simulink model "actuator_control"  (R2016b)
settings: configuration reference "Configuration4khz" (kept outside this file)
values from neighbouring files (symbols this model uses):
  sample_time = 0.0005    [ElmoIncremental.m]
undefined symbols (not defined in the file or in its folder): A_kalman_sea_swing_back, A_kalman_sea_swing_front, A_kalman_swing_load, A_lpf_1to4, A_lpf_dtau, A_lpf_sea_kalman_velocities, B1_lpf_1to4, B1_lpf_dtau, B1_lpf_sea_kalman_velocities, B2_lpf_1to4, B2_lpf_dtau, B2_lpf_sea_kalman_velocities, B_kalman_sea_swing_back, B_kalman_sea_swing_front, B_kalman_swing_load, C_kalman_sea_swing, C_kalman_swing_load, DiscIntNeverNeededParam, Discrete, elmo_sample_time, fdesignblkfcn, gcbh, initial_dx_estimate, j_segments, k_sea_low, kalman_load_to_deflect_transmission, lateral_motor_efficiency, LEG_MTR_GEAR_RATIO, P0_kalman_sea_swing, P0_kalman_swing_load, Q_kalman_load_torque, Q_kalman_rotor_torque, Q_kalman_trunk_torque, R_kalman_absolute_fail, R_kalman_absolute_normal, R_kalman_incremental_loaded, R_kalman_incremental_unloaded, sea_kalman_sample_time, swing_collision_damping_rate, Time
libraries: simulink x17, ctrlSharedLib x8, dsparch4 x5, dspfdesign x1
(part 2 of 3)

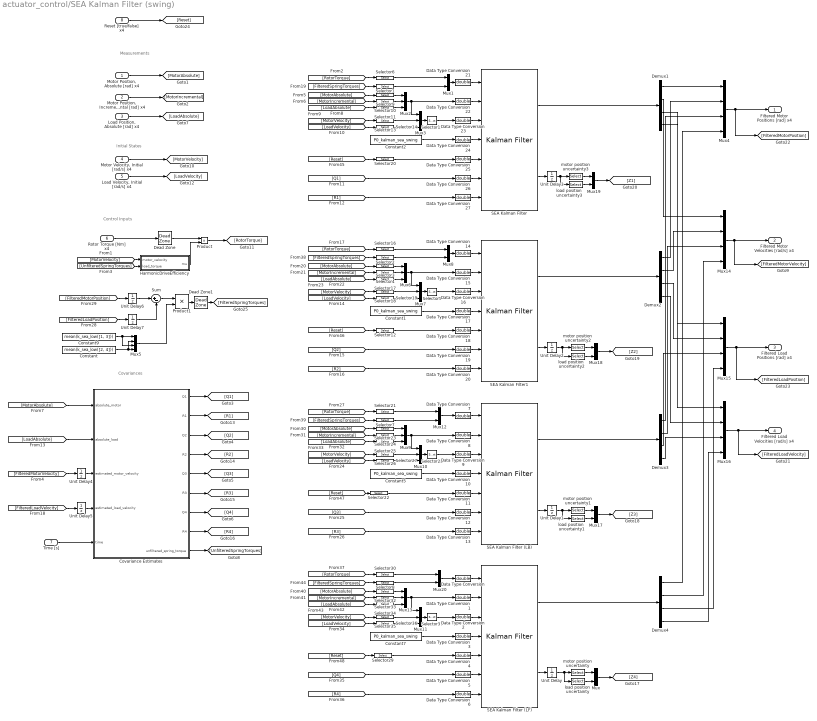
== system actuator_control/SEA Kalman Filter (swing) ==
  note: Measurements
  note: Control Inputs
  note: Initial States
  note: Covariances
  "Motor Position, Absolute [rad] x4" : Inport
  "Motor Position, Incremental [rad] x4" : Inport  Port=2
  "Load Position, Absolute [rad] x4" : Inport  Port=3
  "Motor Velocity, Initial [rad/s] x4" : Inport  Port=4
  "Load Velocity, Initial [rad/s] x4" : Inport  Port=5
  Rotor Torque [Nm] x4 : Inport  Port=6
  Time [s] : Inport  Port=7
  Reset [true/false] x4 : Inport  Port=8
  Constant : Constant  Value=mean(k_sea_low([2, 4]))
  Constant{1..2,5,7} (4 alike) : Constant  Value=P0_kalman_sea_swing
  Constant9 : Constant  Value=mean(k_sea_low([1, 3]))
  Covariance Estimates : MATLAB Function  TreatAsAtomicUnit=on
  Data Type Conversion{,1..27} (28 alike) : DataTypeConversion  OutDataTypeStr=double
  Dead Zone : DeadZone  LowerValue=-30/50  UpperValue=30/50  SaturateOnIntegerOverflow=on
  Dead Zone1 : DeadZone  LowerValue=-2.5  UpperValue=2.5  SaturateOnIntegerOverflow=on
  Demux{1..4} (4 alike) : Demux
  HarmonicDriveEfficiency : MATLAB Function  TreatAsAtomicUnit=on
  Mux{,1,8,12,17..20} (8 alike) : Mux  Inputs=2
  Mux{2..3,6..7,9..11,13} (8 alike) : Mux  Inputs=3
  Mux{4..5,14..16} (5 alike) : Mux
  Product : Product
  Product1 : Product
  SEA Kalman Filter : ctrlSharedLib/Kalman Filter  TimeDomain=Discrete-Time  UseCurrentEstimator=on  ModelSource=Individual A, B, C, D matrices  ModelSourceVariable=A_kf  A=A_kalman_sea_swing_back  B=B_kalman_sea_swing_back  C=C_kalman_sea_swing  D=0  NumberOfStates=2  NumberOfInputs=1  NumberOfOutputs=2  InitialEstimateSource=Input port  X0=initial_dx_estimate  P0=P0_kalman_transverse  UseK=off  UseGH=on  NumberOfProcessNoiseInputs=1  G=G_kalman_sea_swing_back  TimeInvariantG=on  H=0  TimeInvariantH=on  Q=1  TimeInvariantQ=off  R=1  TimeInvariantR=off  N=0  TimeInvariantN=on  AddInputPort=on  AddEnablePort=off  ExternalReset=Rising  OutputEstimatedY=off  OutputP=on  Ts=sea_kalman_sample_time
  SEA Kalman Filter (LB) : ctrlSharedLib/Kalman Filter  TimeDomain=Discrete-Time  UseCurrentEstimator=on  ModelSource=Individual A, B, C, D matrices  ModelSourceVariable=A_kf  A=A_kalman_sea_swing_back  B=B_kalman_sea_swing_back  C=C_kalman_sea_swing  D=0  NumberOfStates=2  NumberOfInputs=1  NumberOfOutputs=2  InitialEstimateSource=Input port  X0=initial_dx_estimate  P0=P0_kalman_transverse  UseK=off  UseGH=on  NumberOfProcessNoiseInputs=1  G=G_kalman_sea_swing_back  TimeInvariantG=on  H=0  TimeInvariantH=on  Q=1  TimeInvariantQ=off  R=1  TimeInvariantR=off  N=0  TimeInvariantN=on  AddInputPort=on  AddEnablePort=off  ExternalReset=Rising  OutputEstimatedY=off  OutputP=on  Ts=sea_kalman_sample_time
  SEA Kalman Filter (LF) : ctrlSharedLib/Kalman Filter  TimeDomain=Discrete-Time  UseCurrentEstimator=on  ModelSource=Individual A, B, C, D matrices  ModelSourceVariable=A_kf  A=A_kalman_sea_swing_front  B=B_kalman_sea_swing_front  C=C_kalman_sea_swing  D=0  NumberOfStates=2  NumberOfInputs=1  NumberOfOutputs=2  InitialEstimateSource=Input port  X0=initial_dx_estimate  P0=P0_kalman_transverse  UseK=off  UseGH=on  NumberOfProcessNoiseInputs=1  G=G_kalman_sea_swing_front  TimeInvariantG=on  H=0  TimeInvariantH=on  Q=1  TimeInvariantQ=off  R=1  TimeInvariantR=off  N=0  TimeInvariantN=on  AddInputPort=on  AddEnablePort=off  ExternalReset=Rising  OutputEstimatedY=off  OutputP=on  Ts=sea_kalman_sample_time
  SEA Kalman Filter1 : ctrlSharedLib/Kalman Filter  TimeDomain=Discrete-Time  UseCurrentEstimator=on  ModelSource=Individual A, B, C, D matrices  ModelSourceVariable=A_kf  A=A_kalman_sea_swing_front  B=B_kalman_sea_swing_front  C=C_kalman_sea_swing  D=0  NumberOfStates=2  NumberOfInputs=1  NumberOfOutputs=2  InitialEstimateSource=Input port  X0=initial_dx_estimate  P0=P0_kalman_transverse  UseK=off  UseGH=on  NumberOfProcessNoiseInputs=1  G=G_kalman_sea_swing_front  TimeInvariantG=on  H=0  TimeInvariantH=on  Q=1  TimeInvariantQ=off  R=1  TimeInvariantR=off  N=0  TimeInvariantN=on  AddInputPort=on  AddEnablePort=off  ExternalReset=Rising  OutputEstimatedY=off  OutputP=on  Ts=sea_kalman_sample_time
  Selector{1,6,9..11,13..14,20} (8 alike) : Selector  InputPortWidth=4  IndexOptions=Index vector (dialog)  Indices=[1]  OutputSizes=1
  Selector{2..4,12,16..19} (8 alike) : Selector  InputPortWidth=4  IndexOptions=Index vector (dialog)  Indices=[2]  OutputSizes=1
  Selector{5,15,28,37} (4 alike) : Selector  InputPortWidth=5  IndexOptions=Index vector (dialog)  Indices=[1 4 3 5]  OutputSizes=1
  Selector{7,21..27} (8 alike) : Selector  InputPortWidth=4  IndexOptions=Index vector (dialog)  Indices=[3]  OutputSizes=1
  Selector{8,29..30,32..36} (8 alike) : Selector  InputPortWidth=4  IndexOptions=Index vector (dialog)  Indices=[4]  OutputSizes=1
  Sum : Sum  Inputs=|+-
  Unit Delay{,1..7} (8 alike) : UnitDelay  SampleTime=-1
  load position uncertainty{,1..3} (4 alike) : Selector  NumberOfDimensions=2  InputPortWidth=2  IndexOptions=Index vector (dialog),Index vector (dialog)  Indices=[3],[3]  OutputSizes=1,1
  motor position uncertainty{,1..3} (4 alike) : Selector  NumberOfDimensions=2  InputPortWidth=2  IndexOptions=Index vector (dialog),Index vector (dialog)  Indices=[1],[1]  OutputSizes=1,1
  Filtered Motor Positions [rad] x4 : Outport
  Filtered Motor Velocities [rad/s] x4 : Outport  Port=2
  Filtered Load Positions [rad] x4 : Outport  Port=3
  Filtered Load Velocities [rad/s] x4 : Outport  Port=4
  wires:
  "Motor Position, Incremental [rad] x4"/1 -> [MotorIncremental]
  "Motor Position, Absolute [rad] x4"/1 -> [MotorAbsolute]
  "Load Position, Absolute [rad] x4"/1 -> [LoadAbsolute]
  Mux2/1 -> Mux3/1, Data Type Conversion22/1
  Selector6/1 -> Mux1/1
  [RotorTorque] -> Selector6/1
  Selector11/1 -> Mux2/3
  Selector10/1 -> Mux2/2
  Selector9/1 -> Mux2/1
  [MotorAbsolute] -> Selector9/1
  [MotorIncremental] -> Selector10/1
  [LoadAbsolute] -> Selector11/1
  "Motor Velocity, Initial [rad/s] x4"/1 -> [MotorVelocity]
  "Load Velocity, Initial [rad/s] x4"/1 -> [LoadVelocity]
  Mux3/1 -> Selector15/1
  [MotorVelocity] -> Selector13/1
  [LoadVelocity] -> Selector14/1
  Selector14/1 -> Mux3/3
  Selector13/1 -> Mux3/2
  Selector15/1 -> Data Type Conversion23/1
  Constant2/1 -> Data Type Conversion24/1
  [Reset] -> Selector20/1
  [R1] -> Data Type Conversion27/1
  [Q1] -> Data Type Conversion26/1
  SEA Kalman Filter/1 -> Demux1/1
  Covariance Estimates/1(Q1) -> [Q1]
  Covariance Estimates/3(Q2) -> [Q2]
  Covariance Estimates/5(Q3) -> [Q3]
  Covariance Estimates/7(Q4) -> [Q4]
  Covariance Estimates/2(R1) -> [R1]
  Covariance Estimates/4(R2) -> [R2]
  Covariance Estimates/6(R3) -> [R3]
  Covariance Estimates/8(R4) -> [R4]
  Mux6/1 -> Data Type Conversion15/1, Mux7/1
  [RotorTorque] -> Selector16/1
  Selector17/1 -> Mux6/3
  Selector4/1 -> Mux6/2
  Selector3/1 -> Mux6/1
  [MotorAbsolute] -> Selector3/1
  [MotorIncremental] -> Selector4/1
  [LoadAbsolute] -> Selector17/1
  Mux7/1 -> Selector5/1
  [MotorVelocity] -> Selector18/1
  [LoadVelocity] -> Selector19/1
  Selector19/1 -> Mux7/3
  Selector18/1 -> Mux7/2
  Selector5/1 -> Data Type Conversion16/1
  Constant1/1 -> Data Type Conversion17/1
  [Reset] -> Selector12/1
  [R2] -> Data Type Conversion20/1
  [Q2] -> Data Type Conversion19/1
  SEA Kalman Filter1/1 -> Demux2/1
  Mux9/1 -> Mux10/1, Data Type Conversion8/1
  [RotorTorque] -> Selector21/1
  Selector25/1 -> Mux9/3
  Selector24/1 -> Mux9/2
  Selector23/1 -> Mux9/1
  [MotorAbsolute] -> Selector23/1
  [MotorIncremental] -> Selector24/1
  [LoadAbsolute] -> Selector25/1
  Mux10/1 -> Selector28/1
  [MotorVelocity] -> Selector26/1
  [LoadVelocity] -> Selector27/1
  Selector27/1 -> Mux10/3
  Selector26/1 -> Mux10/2
  Selector28/1 -> Data Type Conversion9/1
  Constant5/1 -> Data Type Conversion10/1
  [Reset] -> Selector22/1
  [R3] -> Data Type Conversion13/1
  [Q3] -> Data Type Conversion12/1
  SEA Kalman Filter (LB)/1 -> Demux3/1
  Mux13/1 -> Data Type Conversion1/1, Mux11/1
  [RotorTorque] -> Selector30/1
  Selector34/1 -> Mux13/3
  Selector33/1 -> Mux13/2
  Selector32/1 -> Mux13/1
  [MotorAbsolute] -> Selector32/1
  [MotorIncremental] -> Selector33/1
  [LoadAbsolute] -> Selector34/1
  Mux11/1 -> Selector37/1
  [MotorVelocity] -> Selector35/1
  [LoadVelocity] -> Selector36/1
  Selector36/1 -> Mux11/3
  Selector35/1 -> Mux11/2
  Selector37/1 -> Data Type Conversion2/1
  Constant7/1 -> Data Type Conversion3/1
  [Reset] -> Selector29/1
  [R4] -> Data Type Conversion6/1
  [Q4] -> Data Type Conversion5/1
  SEA Kalman Filter (LF)/1 -> Demux4/1
  Demux1/1 -> Mux4/1
  Demux2/1 -> Mux4/2
  Demux3/1 -> Mux4/3
  Demux4/1 -> Mux4/4
  Demux1/2 -> Mux14/1
  Demux2/2 -> Mux14/2
  Demux3/2 -> Mux14/3
  Demux4/2 -> Mux14/4
  Demux1/3 -> Mux15/1
  Demux2/3 -> Mux15/2
  Demux3/3 -> Mux15/3
  Demux4/3 -> Mux15/4
  Demux1/4 -> Mux16/1
  Demux2/4 -> Mux16/2
  Demux3/4 -> Mux16/3
  Demux4/4 -> Mux16/4
  [LoadAbsolute] -> Covariance Estimates/2(absolute_load)
  [MotorAbsolute] -> Covariance Estimates/1(absolute_motor)
  SEA Kalman Filter (LF)/2 -> Unit Delay/1
  motor position uncertainty/1 -> Mux/1
  load position uncertainty/1 -> Mux/2
  Mux/1 -> [Z4]
  SEA Kalman Filter (LB)/2 -> Unit Delay1/1
  motor position uncertainty1/1 -> Mux17/1
  load position uncertainty1/1 -> Mux17/2
  Mux17/1 -> [Z3]
  SEA Kalman Filter1/2 -> Unit Delay2/1
  motor position uncertainty2/1 -> Mux18/1
  load position uncertainty2/1 -> Mux18/2
  Mux18/1 -> [Z2]
  SEA Kalman Filter/2 -> Unit Delay3/1
  motor position uncertainty3/1 -> Mux19/1
  load position uncertainty3/1 -> Mux19/2
  Mux19/1 -> [Z1]
  Unit Delay/1 -> load position uncertainty/1, motor position uncertainty/1
  Unit Delay1/1 -> load position uncertainty1/1, motor position uncertainty1/1
  Unit Delay2/1 -> motor position uncertainty2/1, load position uncertainty2/1
  Unit Delay3/1 -> load position uncertainty3/1, motor position uncertainty3/1
  Data Type Conversion/1 -> SEA Kalman Filter (LF)/1
  Data Type Conversion1/1 -> SEA Kalman Filter (LF)/2
  Data Type Conversion2/1 -> SEA Kalman Filter (LF)/3
  Data Type Conversion3/1 -> SEA Kalman Filter (LF)/4
  Data Type Conversion4/1 -> SEA Kalman Filter (LF)/5
  Data Type Conversion5/1 -> SEA Kalman Filter (LF)/6
  Data Type Conversion6/1 -> SEA Kalman Filter (LF)/7
  Data Type Conversion7/1 -> SEA Kalman Filter (LB)/1
  Data Type Conversion9/1 -> SEA Kalman Filter (LB)/3
  Data Type Conversion8/1 -> SEA Kalman Filter (LB)/2
  Data Type Conversion10/1 -> SEA Kalman Filter (LB)/4
  Data Type Conversion11/1 -> SEA Kalman Filter (LB)/5
  Data Type Conversion13/1 -> SEA Kalman Filter (LB)/7
  Data Type Conversion12/1 -> SEA Kalman Filter (LB)/6
  Data Type Conversion14/1 -> SEA Kalman Filter1/1
  Data Type Conversion15/1 -> SEA Kalman Filter1/2
  Data Type Conversion18/1 -> SEA Kalman Filter1/5
  Data Type Conversion19/1 -> SEA Kalman Filter1/6
  Data Type Conversion16/1 -> SEA Kalman Filter1/3
  Data Type Conversion17/1 -> SEA Kalman Filter1/4
  Data Type Conversion20/1 -> SEA Kalman Filter1/7
  Data Type Conversion21/1 -> SEA Kalman Filter/1
  Data Type Conversion25/1 -> SEA Kalman Filter/5
  Data Type Conversion24/1 -> SEA Kalman Filter/4
  Data Type Conversion23/1 -> SEA Kalman Filter/3
  Data Type Conversion26/1 -> SEA Kalman Filter/6
  Data Type Conversion22/1 -> SEA Kalman Filter/2
  Data Type Conversion27/1 -> SEA Kalman Filter/7
  Mux4/1 -> [FilteredMotorPosition], Filtered Motor Positions [rad] x4/1
  Mux15/1 -> [FilteredLoadPosition], Filtered Load Positions [rad] x4/1
  Mux14/1 -> [FilteredMotorVelocity], Filtered Motor Velocities [rad/s] x4/1
  Mux16/1 -> [FilteredLoadVelocity], Filtered Load Velocities [rad/s] x4/1
  HarmonicDriveEfficiency/1(mu) -> Product/2
  [MotorVelocity] -> HarmonicDriveEfficiency/1(motor_velocity)
  [UnfilteredSpringTorques] -> HarmonicDriveEfficiency/2(load_torque)
  Covariance Estimates/9(unfiltered_spring_torque) -> [UnfilteredSpringTorques]
  Time [s]/1 -> Covariance Estimates/5(time)
  [FilteredMotorVelocity] -> Unit Delay4/1
  [FilteredLoadVelocity] -> Unit Delay5/1
  Unit Delay4/1 -> Covariance Estimates/3(estimated_motor_velocity)
  Unit Delay5/1 -> Covariance Estimates/4(estimated_load_velocity)
  Rotor Torque [Nm] x4/1 -> Dead Zone/1
  Dead Zone/1 -> Product/1
  Mux1/1 -> Data Type Conversion21/1
  [FilteredSpringTorques] -> Selector1/1
  Selector1/1 -> Mux1/2
  [FilteredMotorPosition] -> Unit Delay6/1
  [FilteredLoadPosition] -> Unit Delay7/1
  Constant9/1 -> Mux5/1, Mux5/3
  Constant/1 -> Mux5/2, Mux5/4
  Sum/1 -> Product1/1
  Mux5/1 -> Product1/2
  Product1/1 -> Dead Zone1/1
  [FilteredSpringTorques] -> Selector2/1
  Selector2/1 -> Mux8/2
  Mux8/1 -> Data Type Conversion14/1
  Selector16/1 -> Mux8/1
  [FilteredSpringTorques] -> Selector7/1
  Selector7/1 -> Mux12/2
  Mux12/1 -> Data Type Conversion7/1
  Selector21/1 -> Mux12/1
  [FilteredSpringTorques] -> Selector8/1
  Selector8/1 -> Mux20/2
  Mux20/1 -> Data Type Conversion/1
  Selector30/1 -> Mux20/1
  Unit Delay7/1 -> Sum/2
  Unit Delay6/1 -> Sum/1
  Dead Zone1/1 -> [FilteredSpringTorques]
  Product/1 -> [RotorTorque]
  Reset [true/false] x4/1 -> [Reset]
  Selector12/1 -> Data Type Conversion18/1
  Selector20/1 -> Data Type Conversion25/1
  Selector22/1 -> Data Type Conversion11/1
  Selector29/1 -> Data Type Conversion4/1

== system actuator_control/Select Signal ==
  True/False x4 : Inport
  Signal True x4 : Inport  Port=2
  Signal False x4 : Inport  Port=3
  Demux : Demux
  Demux1 : Demux
  Demux2 : Demux
  Mux : Mux
  Switch{,1..3} (4 alike) : Switch  Criteria=u2 ~= 0
  Selected x4 : Outport
  wires:
  Mux/1 -> Selected x4/1
  True/False x4/1 -> Demux1/1
  Signal True x4/1 -> Demux/1
  Signal False x4/1 -> Demux2/1
  Demux/1 -> Switch/1
  Demux/2 -> Switch1/1
  Demux/3 -> Switch2/1
  Demux/4 -> Switch3/1
  Demux2/1 -> Switch/3
  Demux2/2 -> Switch1/3
  Demux2/3 -> Switch2/3
  Demux2/4 -> Switch3/3
  Demux1/1 -> Switch/2
  Demux1/2 -> Switch1/2
  Demux1/3 -> Switch2/2
  Demux1/4 -> Switch3/2
  Switch/1 -> Mux/1
  Switch1/1 -> Mux/2
  Switch2/1 -> Mux/3
  Switch3/1 -> Mux/4

== system actuator_control/Select Signal1 ==
  True/False x4 : Inport
  Signal True x4 : Inport  Port=2
  Signal False x4 : Inport  Port=3
  Demux : Demux
  Demux1 : Demux
  Demux2 : Demux
  Mux : Mux
  Switch{,1..3} (4 alike) : Switch  Criteria=u2 ~= 0
  Selected x4 : Outport
  wires:
  Switch3/1 -> Mux/4
  Switch2/1 -> Mux/3
  Switch1/1 -> Mux/2
  Switch/1 -> Mux/1
  Demux1/4 -> Switch3/2
  Demux1/3 -> Switch2/2
  Demux1/2 -> Switch1/2
  Demux1/1 -> Switch/2
  Demux2/4 -> Switch3/3
  Demux2/3 -> Switch2/3
  Demux2/2 -> Switch1/3
  Demux2/1 -> Switch/3
  Demux/4 -> Switch3/1
  Demux/3 -> Switch2/1
  Demux/2 -> Switch1/1
  Demux/1 -> Switch/1
  Signal False x4/1 -> Demux2/1
  Signal True x4/1 -> Demux/1
  True/False x4/1 -> Demux1/1
  Mux/1 -> Selected x4/1

== system actuator_control/Select Signal2 ==
  True/False x4 : Inport
  Signal True x4 : Inport  Port=2
  Signal False x4 : Inport  Port=3
  Demux : Demux
  Demux1 : Demux
  Demux2 : Demux
  Mux : Mux
  Switch{,1..3} (4 alike) : Switch  Criteria=u2 ~= 0
  Selected x4 : Outport
  wires:
  Mux/1 -> Selected x4/1
  True/False x4/1 -> Demux1/1
  Signal True x4/1 -> Demux/1
  Signal False x4/1 -> Demux2/1
  Demux/1 -> Switch/1
  Demux/2 -> Switch1/1
  Demux/3 -> Switch2/1
  Demux/4 -> Switch3/1
  Demux2/1 -> Switch/3
  Demux2/2 -> Switch1/3
  Demux2/3 -> Switch2/3
  Demux2/4 -> Switch3/3
  Demux1/1 -> Switch/2
  Demux1/2 -> Switch1/2
  Demux1/3 -> Switch2/2
  Demux1/4 -> Switch3/2
  Switch/1 -> Mux/1
  Switch1/1 -> Mux/2
  Switch2/1 -> Mux/3
  Switch3/1 -> Mux/4

== system actuator_control/Stance or Swing1 ==
  True/False x4 : Inport
  Signal True x4 : Inport  Port=2
  Signal False x4 : Inport  Port=3
  Demux : Demux
  Demux1 : Demux
  Demux2 : Demux
  Mux : Mux
  Switch{,1..3} (4 alike) : Switch  Criteria=u2 ~= 0
  Selected x4 : Outport
  wires:
  Switch3/1 -> Mux/4
  Switch2/1 -> Mux/3
  Switch1/1 -> Mux/2
  Switch/1 -> Mux/1
  Demux1/4 -> Switch3/2
  Demux1/3 -> Switch2/2
  Demux1/2 -> Switch1/2
  Demux1/1 -> Switch/2
  Demux2/4 -> Switch3/3
  Demux2/3 -> Switch2/3
  Demux2/2 -> Switch1/3
  Demux2/1 -> Switch/3
  Demux/4 -> Switch3/1
  Demux/3 -> Switch2/1
  Demux/2 -> Switch1/1
  Demux/1 -> Switch/1
  Signal False x4/1 -> Demux2/1
  Signal True x4/1 -> Demux/1
  True/False x4/1 -> Demux1/1
  Mux/1 -> Selected x4/1

== system actuator_control/Misc/Compare SEA Signals1 ==
  Finite Difference : Inport
  Kalman : Inport  Port=2
  Demux : Demux
  Demux1 : Demux
  Mux{6..9} (4 alike) : Mux  Inputs=2
  RB : Outport
  RF : Outport  Port=2
  LB : Outport  Port=3
  LF : Outport  Port=4
  wires:
  Demux/3 -> Mux8/1
  Demux/2 -> Mux7/1
  Demux1/1 -> Mux6/2
  Demux/1 -> Mux6/1
  Demux/4 -> Mux9/1
  Demux1/4 -> Mux9/2
  Kalman/1 -> Demux1/1
  Demux1/2 -> Mux7/2
  Finite Difference/1 -> Demux/1
  Demux1/3 -> Mux8/2
  Mux6/1 -> RB/1
  Mux7/1 -> RF/1
  Mux9/1 -> LF/1
  Mux8/1 -> LB/1

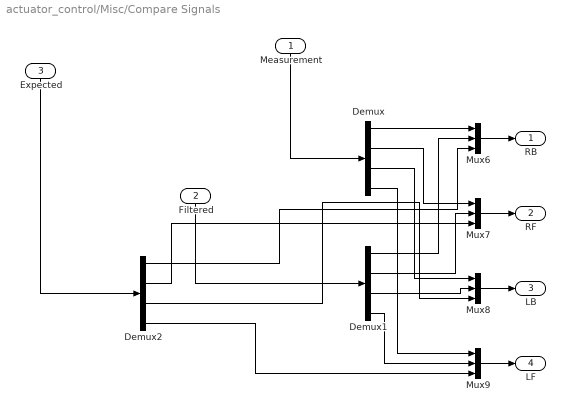
== system actuator_control/Misc/Compare Signals ==
  Measurement : Inport
  Filtered : Inport  Port=2
  Expected : Inport  Port=3
  Demux : Demux
  Demux1 : Demux
  Demux2 : Demux
  Mux{6..9} (4 alike) : Mux  Inputs=3
  RB : Outport
  RF : Outport  Port=2
  LB : Outport  Port=3
  LF : Outport  Port=4
  wires:
  Mux8/1 -> LB/1
  Mux9/1 -> LF/1
  Mux7/1 -> RF/1
  Mux6/1 -> RB/1
  Demux1/3 -> Mux8/2
  Measurement/1 -> Demux/1
  Demux1/2 -> Mux7/2
  Filtered/1 -> Demux1/1
  Demux1/4 -> Mux9/2
  Demux/4 -> Mux9/1
  Demux/1 -> Mux6/1
  Demux1/1 -> Mux6/2
  Demux/2 -> Mux7/1
  Demux/3 -> Mux8/1
  Expected/1 -> Demux2/1
  Demux2/1 -> Mux6/3
  Demux2/2 -> Mux7/3
  Demux2/3 -> Mux8/3
  Demux2/4 -> Mux9/3

== system actuator_control/Misc/Compare Torque Derivative Signals ==
  Measured : Inport
  Filtered : Inport  Port=2
  Expected : Inport  Port=3
  Demux : Demux
  Demux1 : Demux
  Demux2 : Demux
  Mux{6..9} (4 alike) : Mux  Inputs=3
  RB : Outport
  RF : Outport  Port=2
  LB : Outport  Port=3
  LF : Outport  Port=4
  wires:
  Demux2/4 -> Mux9/3
  Demux2/3 -> Mux8/3
  Demux2/2 -> Mux7/3
  Demux2/1 -> Mux6/3
  Expected/1 -> Demux2/1
  Demux/3 -> Mux8/1
  Demux/2 -> Mux7/1
  Demux1/1 -> Mux6/2
  Demux/1 -> Mux6/1
  Demux/4 -> Mux9/1
  Demux1/4 -> Mux9/2
  Filtered/1 -> Demux1/1
  Demux1/2 -> Mux7/2
  Measured/1 -> Demux/1
  Demux1/3 -> Mux8/2
  Mux6/1 -> RB/1
  Mux7/1 -> RF/1
  Mux9/1 -> LF/1
  Mux8/1 -> LB/1

== system actuator_control/Misc/Contact Velocities ==
  Contact [1/0] x4 : Inport
  Velocities [rad/s] x4 : Inport  Port=2
  Demux : Demux
  Demux1 : Demux
  Mux : Mux
  Velocity on Contact : Subsystem
  Velocity on Contact1 : Subsystem
  Velocity on Contact2 : Subsystem
  Velocity on Contact3 : Subsystem
  Contact Velocities [rad/s] x4 : Outport
  wires:
  Mux/1 -> Contact Velocities [rad/s] x4/1
  Demux/2 -> Velocity on Contact1/Trigger
  Velocity on Contact/1(out) -> Mux/1
  Contact [1/0] x4/1 -> Demux/1
  Velocity on Contact1/1(out) -> Mux/2
  Demux/3 -> Velocity on Contact2/Trigger
  Demux/4 -> Velocity on Contact3/Trigger
  Demux/1 -> Velocity on Contact/Trigger
  Velocity on Contact3/1(out) -> Mux/4
  Velocity on Contact2/1(out) -> Mux/3
  Velocities [rad/s] x4/1 -> Demux1/1
  Demux1/1 -> Velocity on Contact/1(in)
  Demux1/2 -> Velocity on Contact1/1(in)
  Demux1/3 -> Velocity on Contact2/1(in)
  Demux1/4 -> Velocity on Contact3/1(in)

== system actuator_control/Misc/Expected Forces on Foot ==
  R/L Leg Length [m] x2 : Inport
  R/L Leg Width [m] x2 : Inport  Port=2
  Torques on Load [Nm] x4 : Inport  Port=3
  Divide : Product  Inputs=/*
  Divide1 : Product  Inputs=/*
  Gain3 : Gain  Gain=-1
  Gain6 : Gain  Gain=-1
  Selector2 : Selector  InputPortWidth=4  IndexOptions=Index vector (dialog)  Indices=[1 3]  OutputSizes=1
  Selector7 : Selector  InputPortWidth=4  IndexOptions=Index vector (dialog)  Indices=[2 4]  OutputSizes=1
  Sum5 : Sum  Inputs=|-+
  Sum6 : Sum  Inputs=++|
  R/L Orthogonal Force [N] x2 : Outport
  R/L Axial Force [N] x2 : Outport  Port=2
  wires:
  Gain6/1 -> R/L Orthogonal Force [N] x2/1
  Gain3/1 -> R/L Axial Force [N] x2/1
  Sum5/1 -> Divide1/2
  Selector7/1 -> Sum6/2, Sum5/2
  Sum6/1 -> Divide/2
  Selector2/1 -> Sum5/1, Sum6/1
  Divide1/1 -> Gain3/1
  Torques on Load [Nm] x4/1 -> Selector2/1, Selector7/1
  R/L Leg Width [m] x2/1 -> Divide1/1
  R/L Leg Length [m] x2/1 -> Divide/1
  Divide/1 -> Gain6/1

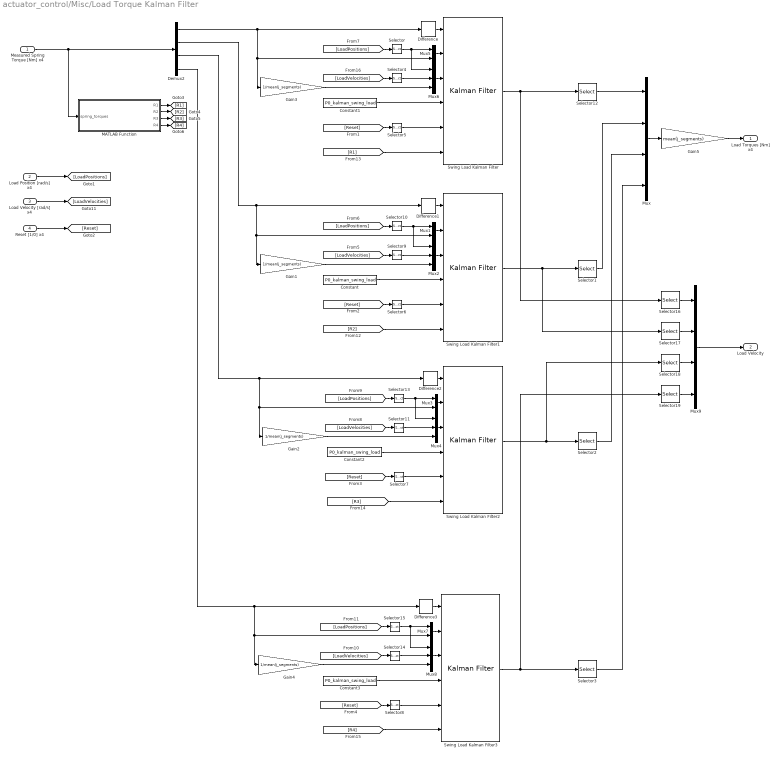
== system actuator_control/Misc/Load Torque Kalman Filter ==
  Measured Spring Torque [Nm] x4 : Inport
  Load Position [rad/s] x4 : Inport  Port=2
  Load Velocity [rad/s] x4 : Inport  Port=3
  Reset [1/0] x4 : Inport  Port=4
  Constant{,1..3} (4 alike) : Constant  Value=P0_kalman_swing_load
  Demux2 : Demux
  Difference{,1..3} (4 alike) : simulink/Discrete/Difference  ICPrevInput=0.0  InputProcessing=Inherited  OutMin=[]  OutMax=[]  OutDataType=fixdt(1, 16)  OutScaling=2^-10  DoSatur=off
  Gain{1..4} (4 alike) : Gain  Gain=1/mean(j_segments)
  Gain5 : Gain  Gain=mean(j_segments)
  MATLAB Function : MATLAB Function  TreatAsAtomicUnit=on
  Mux : Mux
  Mux{1,3,5,7} (4 alike) : Mux  Inputs=2
  Mux{2,4,6,8} (4 alike) : Mux  Inputs=3
  Mux9 : Mux
  Selector : Selector  InputPortWidth=4  IndexOptions=Index vector (dialog)  Indices=[1]  OutputSizes=1
  Selector{1..3,12} (4 alike) : Selector  InputPortWidth=3  IndexOptions=Index vector (dialog)  Indices=[3]  OutputSizes=1
  Selector10 : Selector  InputPortWidth=4  IndexOptions=Index vector (dialog)  Indices=[2]  OutputSizes=1
  Selector11 : Selector  InputPortWidth=4  IndexOptions=Index vector (dialog)  Indices=[3]  OutputSizes=1
  Selector13 : Selector  InputPortWidth=4  IndexOptions=Index vector (dialog)  Indices=[3]  OutputSizes=1
  Selector14 : Selector  InputPortWidth=4  IndexOptions=Index vector (dialog)  Indices=[4]  OutputSizes=1
  Selector15 : Selector  InputPortWidth=4  IndexOptions=Index vector (dialog)  Indices=[4]  OutputSizes=1
  Selector{16..19} (4 alike) : Selector  InputPortWidth=3  IndexOptions=Index vector (dialog)  Indices=[2]  OutputSizes=1
  Selector4 : Selector  InputPortWidth=4  IndexOptions=Index vector (dialog)  Indices=[1]  OutputSizes=1
  Selector5 : Selector  InputPortWidth=4  IndexOptions=Index vector (dialog)  Indices=[1]  OutputSizes=1
  Selector6 : Selector  InputPortWidth=4  IndexOptions=Index vector (dialog)  Indices=[2]  OutputSizes=1
  Selector7 : Selector  InputPortWidth=4  IndexOptions=Index vector (dialog)  Indices=[3]  OutputSizes=1
  Selector8 : Selector  InputPortWidth=4  IndexOptions=Index vector (dialog)  Indices=[4]  OutputSizes=1
  Selector9 : Selector  InputPortWidth=4  IndexOptions=Index vector (dialog)  Indices=[2]  OutputSizes=1
  Swing Load Kalman Filter{,1..3} (4 alike) : ctrlSharedLib/Kalman Filter  TimeDomain=Discrete-Time  UseCurrentEstimator=on  ModelSource=Individual A, B, C, D matrices  ModelSourceVariable=A_kf  A=A_kalman_swing_load  B=B_kalman_swing_load  C=C_kalman_swing_load  D=0  NumberOfStates=2  NumberOfInputs=1  NumberOfOutputs=2  InitialEstimateSource=Input port  X0=initial_dx_estimate  P0=P0_kalman_transverse  UseK=off  UseGH=on  NumberOfProcessNoiseInputs=1  G=G_kalman_swing_load  TimeInvariantG=on  H=0  TimeInvariantH=on  Q=Q_kalman_SEA_torque_difference  TimeInvariantQ=on  R=1  TimeInvariantR=off  N=0  TimeInvariantN=on  AddInputPort=on  AddEnablePort=off  ExternalReset=Rising  OutputEstimatedY=off  OutputP=off  Ts=sample_time
  Load Torques [Nm] x4 : Outport
  Load Velocity : Outport  Port=2
  wires:
  Mux6/1 -> Swing Load Kalman Filter/3
  Mux5/1 -> Swing Load Kalman Filter/2
  Difference/1 -> Swing Load Kalman Filter/1
  Demux2/1 -> Gain3/1, Mux5/2, Difference/1
  Swing Load Kalman Filter/1 -> Selector16/1, Selector12/1
  Selector12/1 -> Mux/1
  Mux2/1 -> Swing Load Kalman Filter1/3
  Mux1/1 -> Swing Load Kalman Filter1/2
  Difference1/1 -> Swing Load Kalman Filter1/1
  Demux2/2 -> Gain1/1, Mux1/2, Difference1/1
  Gain1/1 -> Mux2/3
  Mux4/1 -> Swing Load Kalman Filter2/3
  Mux3/1 -> Swing Load Kalman Filter2/2
  Difference2/1 -> Swing Load Kalman Filter2/1
  Demux2/3 -> Difference2/1, Mux3/2, Gain2/1
  Gain2/1 -> Mux4/3
  Mux8/1 -> Swing Load Kalman Filter3/3
  Mux7/1 -> Swing Load Kalman Filter3/2
  Difference3/1 -> Swing Load Kalman Filter3/1
  Demux2/4 -> Difference3/1, Mux7/2, Gain4/1
  Gain4/1 -> Mux8/3
  Swing Load Kalman Filter1/1 -> Selector17/1, Selector1/1
  Swing Load Kalman Filter3/1 -> Selector19/1, Selector3/1
  Swing Load Kalman Filter2/1 -> Selector18/1, Selector2/1
  Mux/1 -> Gain5/1
  Selector1/1 -> Mux/2
  Selector2/1 -> Mux/3
  Selector3/1 -> Mux/4
  Reset [1/0] x4/1 -> [Reset]
  Load Velocity [rad/s] x4/1 -> [LoadVelocities]
  Measured Spring Torque [Nm] x4/1 -> MATLAB Function/1(spring_torques), Demux2/1
  Gain5/1 -> Load Torques [Nm] x4/1
  Gain3/1 -> Mux6/3
  Load Position [rad/s] x4/1 -> [LoadPositions]
  [LoadPositions] -> Selector/1
  [LoadVelocities] -> Selector4/1
  Selector/1 -> Mux6/1, Mux5/1
  Selector4/1 -> Mux6/2
  [Reset] -> Selector5/1
  Selector5/1 -> Swing Load Kalman Filter/5
  [Reset] -> Selector6/1
  Selector6/1 -> Swing Load Kalman Filter1/5
  [Reset] -> Selector7/1
  Selector7/1 -> Swing Load Kalman Filter2/5
  [Reset] -> Selector8/1
  Selector8/1 -> Swing Load Kalman Filter3/5
  [LoadVelocities] -> Selector9/1
  [LoadPositions] -> Selector10/1
  [LoadVelocities] -> Selector11/1
  [LoadPositions] -> Selector13/1
  [LoadVelocities] -> Selector14/1
  [LoadPositions] -> Selector15/1
  Selector15/1 -> Mux8/1, Mux7/1
  Selector13/1 -> Mux4/1, Mux3/1
  Selector11/1 -> Mux4/2
  Selector14/1 -> Mux8/2
  Selector9/1 -> Mux2/2
  Selector10/1 -> Mux2/1, Mux1/1
  Constant/1 -> Swing Load Kalman Filter1/4
  MATLAB Function/1(R1) -> [R1]
  MATLAB Function/2(R2) -> [R2]
  MATLAB Function/3(R3) -> [R3]
  MATLAB Function/4(R4) -> [R4]
  [R2] -> Swing Load Kalman Filter1/6
  [R1] -> Swing Load Kalman Filter/6
  Constant1/1 -> Swing Load Kalman Filter/4
  [R3] -> Swing Load Kalman Filter2/6
  Constant2/1 -> Swing Load Kalman Filter2/4
  Constant3/1 -> Swing Load Kalman Filter3/4
  [R4] -> Swing Load Kalman Filter3/6
  Mux9/1 -> Load Velocity/1
  Selector16/1 -> Mux9/1
  Selector17/1 -> Mux9/2
  Selector18/1 -> Mux9/3
  Selector19/1 -> Mux9/4

== system actuator_control/Misc/Lowpass Filter ==
  In : Inport
  Generated Filter Block : dsparch4/Biquad Filter  Tag=BlockMethodSubSystem  IIRFiltStruct=Direct form II  CoeffSource=Specify via dialog  BiQuadCoeffs=[1.0054190789171848 -2 1.0054190789171853 1 -1.9557970115108714 0.95685429506963915]  a0Flag=Warning  IC=0  ICnum=0  ICden=0  denAccumFracLength=30  denProdOutputFracLength=30  secondMemoryFracLength=15  roundingMode=Floor  overflowMode=off  ScaleValues=[0.0010519560093213882;92.733879468734756]  optimizeScaleValues=off  ScaleValueMode=Specify via input port (g)  scaleValueFracLength=14  FilterSource=Specify via dialog  FilterObject=Hm_biquad
  Out : Outport
  wires:
  Generated Filter Block/1 -> Out/1
  In/1 -> Generated Filter Block/1

== system actuator_control/Misc/Lowpass Filter1 ==
  In : Inport
  Generated Filter Block : dsparch4/Biquad Filter  Tag=BlockMethodSubSystem  IIRFiltStruct=Direct form II  CoeffSource=Specify via dialog  BiQuadCoeffs=[1.0054190789171848 -2 1.0054190789171853 1 -1.9557970115108714 0.95685429506963915]  a0Flag=Warning  IC=0  ICnum=0  ICden=0  denAccumFracLength=30  denProdOutputFracLength=30  secondMemoryFracLength=15  roundingMode=Floor  overflowMode=off  ScaleValues=[0.0010519560093213882;92.733879468734756]  optimizeScaleValues=off  ScaleValueMode=Specify via input port (g)  scaleValueFracLength=14  FilterSource=Specify via dialog  FilterObject=Hm_biquad
  Out : Outport
  wires:
  In/1 -> Generated Filter Block/1
  Generated Filter Block/1 -> Out/1

== system actuator_control/Misc/Lowpass Filter2 ==
  In : Inport
  Generated Filter Block : dsparch4/Biquad Filter  Tag=BlockMethodSubSystem  IIRFiltStruct=Direct form II  CoeffSource=Specify via dialog  BiQuadCoeffs=[0.42638734887522584 0.71004939850960869 0.42638734887522595 1 0.054295561672899631 0.19751119790393634]  a0Flag=Warning  IC=0  ICnum=0  ICden=0  denAccumFracLength=30  denProdOutputFracLength=30  secondMemoryFracLength=15  roundingMode=Floor  overflowMode=off  ScaleValues=[0.80099018345858064;1]  optimizeScaleValues=off  ScaleValueMode=Specify via input port (g)  scaleValueFracLength=14  FilterSource=Specify via dialog  FilterObject=Hm_biquad
  Out : Outport
  wires:
  In/1 -> Generated Filter Block/1
  Generated Filter Block/1 -> Out/1

== system actuator_control/Misc/Lowpass Filter5 ==
  In : Inport
  Generated Filter Block : dsparch4/Biquad Filter  Tag=BlockMethodSubSystem  IIRFiltStruct=Direct form II  CoeffSource=Specify via dialog  BiQuadCoeffs=[1.0054190789171848 -2 1.0054190789171853 1 -1.9557970115108714 0.95685429506963915]  a0Flag=Warning  IC=0  ICnum=0  ICden=0  denAccumFracLength=30  denProdOutputFracLength=30  secondMemoryFracLength=15  roundingMode=Floor  overflowMode=off  ScaleValues=[0.0010519560093213882;92.733879468734756]  optimizeScaleValues=off  ScaleValueMode=Specify via input port (g)  scaleValueFracLength=14  FilterSource=Specify via dialog  FilterObject=Hm_biquad
  Out : Outport
  wires:
  In/1 -> Generated Filter Block/1
  Generated Filter Block/1 -> Out/1

== system actuator_control/Misc/Lowpass Filter6 ==
  In : Inport
  Generated Filter Block : dsparch4/Biquad Filter  Tag=BlockMethodSubSystem  IIRFiltStruct=Direct form II  CoeffSource=Specify via dialog  BiQuadCoeffs=[1.0054190789171848 -2 1.0054190789171853 1 -1.9557970115108714 0.95685429506963915]  a0Flag=Warning  IC=0  ICnum=0  ICden=0  denAccumFracLength=30  denProdOutputFracLength=30  secondMemoryFracLength=15  roundingMode=Floor  overflowMode=off  ScaleValues=[0.0010519560093213882;92.733879468734756]  optimizeScaleValues=off  ScaleValueMode=Specify via input port (g)  scaleValueFracLength=14  FilterSource=Specify via dialog  FilterObject=Hm_biquad
  Out : Outport
  wires:
  Generated Filter Block/1 -> Out/1
  In/1 -> Generated Filter Block/1

== system actuator_control/Misc/Measured Forces on Foot ==
  R/L Leg Length [m] x2 : Inport
  R/L Leg Width [m] x2 : Inport  Port=2
  Torques on Load [Nm] x4 : Inport  Port=3
  Divide : Product  Inputs=/*
  Divide1 : Product  Inputs=/*
  Gain3 : Gain  Gain=-1
  Gain6 : Gain  Gain=-1
  Selector2 : Selector  InputPortWidth=4  IndexOptions=Index vector (dialog)  Indices=[1 3]  OutputSizes=1
  Selector7 : Selector  InputPortWidth=4  IndexOptions=Index vector (dialog)  Indices=[2 4]  OutputSizes=1
  Sum5 : Sum  Inputs=|-+
  Sum6 : Sum  Inputs=++|
  R/L Orthogonal Force [N] x2 : Outport
  R/L Axial Force [N] x2 : Outport  Port=2
  wires:
  Divide/1 -> Gain6/1
  R/L Leg Length [m] x2/1 -> Divide/1
  R/L Leg Width [m] x2/1 -> Divide1/1
  Torques on Load [Nm] x4/1 -> Selector7/1, Selector2/1
  Divide1/1 -> Gain3/1
  Selector2/1 -> Sum6/1, Sum5/1
  Sum6/1 -> Divide/2
  Selector7/1 -> Sum5/2, Sum6/2
  Sum5/1 -> Divide1/2
  Gain3/1 -> R/L Axial Force [N] x2/1
  Gain6/1 -> R/L Orthogonal Force [N] x2/1

== system actuator_control/Misc/Timers ==
  Start [1/0] x4 : Inport
  Time [s] : Inport  Port=2
  Demux : Demux
  Mux : Mux
  Sum{8..11} (4 alike) : Sum  Inputs=|-+
  Time on Contact : Subsystem
  Time on Contact1 : Subsystem
  Time on Contact2 : Subsystem
  Time on Contact3 : Subsystem
  Timer [s] x4 : Outport
  wires:
  Sum10/1 -> Mux/3
  Sum11/1 -> Mux/4
  Demux/1 -> Time on Contact/Trigger
  Demux/4 -> Time on Contact3/Trigger
  Demux/3 -> Time on Contact2/Trigger
  Time on Contact3/1(out) -> Sum11/1
  Sum9/1 -> Mux/2
  Start [1/0] x4/1 -> Demux/1
  Sum8/1 -> Mux/1
  Time on Contact1/1(out) -> Sum9/1
  Demux/2 -> Time on Contact1/Trigger
  Time [s]/1 -> Time on Contact3/1(in), Time on Contact2/1(in), Time on Contact1/1(in), Time on Contact/1(in), Sum8/2, Sum9/2, Sum11/2, Sum10/2
  Mux/1 -> Timer [s] x4/1
  Time on Contact2/1(out) -> Sum10/1
  Time on Contact/1(out) -> Sum8/1

== system actuator_control/SEA Controller (Velocity Based)/Compare Signals2 ==
  1 : Inport
  2 : Inport  Port=2
  Demux : Demux
  Demux1 : Demux
  Mux{6..9} (4 alike) : Mux  Inputs=2
  RB : Outport
  RF : Outport  Port=2
  LB : Outport  Port=3
  LF : Outport  Port=4
  wires:
  Demux/3 -> Mux8/1
  Demux/2 -> Mux7/1
  Demux1/1 -> Mux6/2
  Demux/1 -> Mux6/1
  Demux/4 -> Mux9/1
  Demux1/4 -> Mux9/2
  2/1 -> Demux1/1
  Demux1/2 -> Mux7/2
  1/1 -> Demux/1
  Demux1/3 -> Mux8/2
  Mux6/1 -> RB/1
  Mux7/1 -> RF/1
  Mux9/1 -> LF/1
  Mux8/1 -> LB/1

== system actuator_control/SEA Controller (Velocity Based)/Integrator ==
  Signal : Inport
  Reset [1/0] : Inport  Port=2
  Demux : Demux
  Demux1 : Demux
  Discrete-Time Integrator{,1..3} (4 alike) : DiscreteIntegrator  ExternalReset=rising  InitialConditionSetting=State (most efficient)  SampleTime=elmo_sample_time  LimitOutput=on  UpperSaturationLimit=1  LowerSaturationLimit=-1  ICPrevOutput=DiscIntNeverNeededParam  ICPrevScaledInput=DiscIntNeverNeededParam
  Mux : Mux
  Integrated : Outport
  wires:
  Demux/4 -> Discrete-Time Integrator3/1
  Demux/3 -> Discrete-Time Integrator2/1
  Demux/2 -> Discrete-Time Integrator1/1
  Demux/1 -> Discrete-Time Integrator/1
  Demux1/1 -> Discrete-Time Integrator/2
  Demux1/2 -> Discrete-Time Integrator1/2
  Demux1/3 -> Discrete-Time Integrator2/2
  Demux1/4 -> Discrete-Time Integrator3/2
  Discrete-Time Integrator3/1 -> Mux/4
  Discrete-Time Integrator2/1 -> Mux/3
  Discrete-Time Integrator1/1 -> Mux/2
  Mux/1 -> Integrated/1
  Reset [1/0]/1 -> Demux1/1
  Discrete-Time Integrator/1 -> Mux/1
  Signal/1 -> Demux/1

== system actuator_control/SEA Controller (Velocity Based)/Lowpass Filter ==
  In : Inport
  Generated Filter Block : DiscreteFir  Tag=BlockMethodSubSystem  Coefficients=[-0.04990855361244094 -0.0010461181532544423 -0.0010107744805273023 -0.00095218248250663988 -0.00085849397163504759 -0.00074175367502442866 -0.00058718772776830946 -0.00041184474721322643 -0.00019652887760975509 4.1532722907783075e-05 0.00031999675256174498 0.00061963547362796486 0.00095907702319196237 0.0013114899691414792 0.0017077848126334939 0.0021254626826913022 0.0025760447586962117 0.0030487109199885914 0.0035497166866013206 0.0040832493046027646 0.0046307261794588678 0.0051947242056444003 0.0057923012727255181 0.0063989592738492437 0.0070358610723892474 0.0076729710874219904 0.0083378124160072738 0.0089921015506421835 0.0096759335261809524 0.010331908705729947 0.011024573190749414 0.011633575605025979 0.012404292046454947 0.013110276864067787 0.013752343250190606 0.01444307115793151 0.015092411392359124 0.015755931236486116 0.01638320562971788 0.017012416656076532 0.017610586760412175 0.018198786428169338 0.018753273958556273 0.019289760931779823 0.01978959816621716 0.020267409454217542 0.020714123209904678 0.02112524451621629 0.021506539266400629 0.021843487024455384 0.022166915431959651 0.022425498521847217 0.02263611511837274 0.022838689821158754 0.022982920388946775 0.023100208768407095 0.023159386359289921 0.023188270363550461 0.023159386359289921 0.023100208768407095 0.022982920388946775 0.022838689821158754 0.02263611511837274 0.022425498521847217 0.022166915431959651 0.021843487024455384 0.021506539266400629 0.02112524451621629 0.020714123209904678 0.020267409454217542 0.01978959816621716 0.019289760931779823 0.018753273958556273 0.018198786428169338 0.017610586760412175 0.017012416656076532 0.01638320562971788 0.015755931236486116 0.015092411392359124 0.01444307115793151 0.013752343250190606 0.013110276864067787 0.012404292046454947 0.011633575605025979 0.011024573190749414 0.010331908705729947 0.0096759335261809524 0.0089921015506421835 0.0083378124160072738 0.0076729710874219904 0.0070358610723892474 0.0063989592738492437 0.0057923012727255181 0.0051947242056444003 0.0046307261794588678 0.0040832493046027646 0.0035497166866013206 0.0030487109199885914 0.0025760447586962117 0.0021254626826913022 0.0017077848126334939 0.0013114899691414792 0.00095907702319196237 0.00061963547362796486 0.00031999675256174498 4.1532722907783075e-05 -0.00019652887760975509 -0.00041184474721322643 -0.00058718772776830946 -0.00074175367502442866 -0.00085849397163504759 -0.00095218248250663988 -0.0010107744805273023 -0.0010461181532544423 -0.04990855361244094]
  Out : Outport
  wires:
  Generated Filter Block/1 -> Out/1
  In/1 -> Generated Filter Block/1

== system actuator_control/SEA Controller (Velocity Based)/Lowpass Filter (30 pass, 60 stop) ==
  In : Inport
  Generated Filter Block : DiscreteFir  Tag=BlockMethodSubSystem  Coefficients=[-0.04990855361244094 -0.0010461181532544423 -0.0010107744805273023 -0.00095218248250663988 -0.00085849397163504759 -0.00074175367502442866 -0.00058718772776830946 -0.00041184474721322643 -0.00019652887760975509 4.1532722907783075e-05 0.00031999675256174498 0.00061963547362796486 0.00095907702319196237 0.0013114899691414792 0.0017077848126334939 0.0021254626826913022 0.0025760447586962117 0.0030487109199885914 0.0035497166866013206 0.0040832493046027646 0.0046307261794588678 0.0051947242056444003 0.0057923012727255181 0.0063989592738492437 0.0070358610723892474 0.0076729710874219904 0.0083378124160072738 0.0089921015506421835 0.0096759335261809524 0.010331908705729947 0.011024573190749414 0.011633575605025979 0.012404292046454947 0.013110276864067787 0.013752343250190606 0.01444307115793151 0.015092411392359124 0.015755931236486116 0.01638320562971788 0.017012416656076532 0.017610586760412175 0.018198786428169338 0.018753273958556273 0.019289760931779823 0.01978959816621716 0.020267409454217542 0.020714123209904678 0.02112524451621629 0.021506539266400629 0.021843487024455384 0.022166915431959651 0.022425498521847217 0.02263611511837274 0.022838689821158754 0.022982920388946775 0.023100208768407095 0.023159386359289921 0.023188270363550461 0.023159386359289921 0.023100208768407095 0.022982920388946775 0.022838689821158754 0.02263611511837274 0.022425498521847217 0.022166915431959651 0.021843487024455384 0.021506539266400629 0.02112524451621629 0.020714123209904678 0.020267409454217542 0.01978959816621716 0.019289760931779823 0.018753273958556273 0.018198786428169338 0.017610586760412175 0.017012416656076532 0.01638320562971788 0.015755931236486116 0.015092411392359124 0.01444307115793151 0.013752343250190606 0.013110276864067787 0.012404292046454947 0.011633575605025979 0.011024573190749414 0.010331908705729947 0.0096759335261809524 0.0089921015506421835 0.0083378124160072738 0.0076729710874219904 0.0070358610723892474 0.0063989592738492437 0.0057923012727255181 0.0051947242056444003 0.0046307261794588678 0.0040832493046027646 0.0035497166866013206 0.0030487109199885914 0.0025760447586962117 0.0021254626826913022 0.0017077848126334939 0.0013114899691414792 0.00095907702319196237 0.00061963547362796486 0.00031999675256174498 4.1532722907783075e-05 -0.00019652887760975509 -0.00041184474721322643 -0.00058718772776830946 -0.00074175367502442866 -0.00085849397163504759 -0.00095218248250663988 -0.0010107744805273023 -0.0010461181532544423 -0.04990855361244094]
  Out : Outport
  wires:
  In/1 -> Generated Filter Block/1
  Generated Filter Block/1 -> Out/1

== system actuator_control/Misc/Contact Velocities/Velocity on Contact ==
  in : Inport
  Trigger : TriggerPort  VariantControl=Variant  ShowOutputPort=on  PortDimensions=1
  Subsystem : Subsystem
  out : Outport
  wires:
  Trigger/1 -> Subsystem/Enable
  Subsystem/1(out) -> out/1
  in/1 -> Subsystem/1(in)

== system actuator_control/Misc/Contact Velocities/Velocity on Contact1 ==
  in : Inport
  Trigger : TriggerPort  VariantControl=Variant  ShowOutputPort=on  PortDimensions=1
  Subsystem : Subsystem
  out : Outport
  wires:
  in/1 -> Subsystem/1(in)
  Subsystem/1(out) -> out/1
  Trigger/1 -> Subsystem/Enable

== system actuator_control/Misc/Contact Velocities/Velocity on Contact2 ==
  in : Inport
  Trigger : TriggerPort  VariantControl=Variant  ShowOutputPort=on  PortDimensions=1
  Subsystem : Subsystem
  out : Outport
  wires:
  in/1 -> Subsystem/1(in)
  Subsystem/1(out) -> out/1
  Trigger/1 -> Subsystem/Enable

== system actuator_control/Misc/Contact Velocities/Velocity on Contact3 ==
  in : Inport
  Trigger : TriggerPort  VariantControl=Variant  ShowOutputPort=on  PortDimensions=1
  Subsystem : Subsystem
  out : Outport
  wires:
  Trigger/1 -> Subsystem/Enable
  Subsystem/1(out) -> out/1
  in/1 -> Subsystem/1(in)

== system actuator_control/Misc/Timers/Time on Contact ==
  in : Inport
  Trigger : TriggerPort  VariantControl=Variant  ShowOutputPort=on  PortDimensions=1
  Subsystem : Subsystem
  out : Outport
  wires:
  in/1 -> Subsystem/1(in)
  Subsystem/1(out) -> out/1
  Trigger/1 -> Subsystem/Enable

== system actuator_control/Misc/Timers/Time on Contact1 ==
  in : Inport
  Trigger : TriggerPort  VariantControl=Variant  ShowOutputPort=on  PortDimensions=1
  Subsystem : Subsystem
  out : Outport
  wires:
  Trigger/1 -> Subsystem/Enable
  Subsystem/1(out) -> out/1
  in/1 -> Subsystem/1(in)

== system actuator_control/Misc/Timers/Time on Contact2 ==
  in : Inport
  Trigger : TriggerPort  VariantControl=Variant  ShowOutputPort=on  PortDimensions=1
  Subsystem : Subsystem
  out : Outport
  wires:
  Trigger/1 -> Subsystem/Enable
  Subsystem/1(out) -> out/1
  in/1 -> Subsystem/1(in)

== system actuator_control/Misc/Timers/Time on Contact3 ==
  in : Inport
  Trigger : TriggerPort  VariantControl=Variant  ShowOutputPort=on  PortDimensions=1
  Subsystem : Subsystem
  out : Outport
  wires:
  in/1 -> Subsystem/1(in)
  Subsystem/1(out) -> out/1
  Trigger/1 -> Subsystem/Enable

== system actuator_control/Misc/Contact Velocities/Velocity on Contact/Subsystem ==
  in : Inport
  Enable : EnablePort
  out : Outport
  wires:
  in/1 -> out/1

== system actuator_control/Misc/Contact Velocities/Velocity on Contact1/Subsystem ==
  in : Inport
  Enable : EnablePort
  out : Outport
  wires:
  in/1 -> out/1

== system actuator_control/Misc/Contact Velocities/Velocity on Contact2/Subsystem ==
  in : Inport
  Enable : EnablePort
  out : Outport
  wires:
  in/1 -> out/1

== system actuator_control/Misc/Contact Velocities/Velocity on Contact3/Subsystem ==
  in : Inport
  Enable : EnablePort
  out : Outport
  wires:
  in/1 -> out/1

== system actuator_control/Misc/Timers/Time on Contact/Subsystem ==
  in : Inport
  Enable : EnablePort
  out : Outport
  wires:
  in/1 -> out/1

== system actuator_control/Misc/Timers/Time on Contact1/Subsystem ==
  in : Inport
  Enable : EnablePort
  out : Outport
  wires:
  in/1 -> out/1

== system actuator_control/Misc/Timers/Time on Contact2/Subsystem ==
  in : Inport
  Enable : EnablePort
  out : Outport
  wires:
  in/1 -> out/1

== system actuator_control/Misc/Timers/Time on Contact3/Subsystem ==
  in : Inport
  Enable : EnablePort
  out : Outport
  wires:
  in/1 -> out/1

== matlab function actuator_control/Misc/Load Torque Kalman Filter/MATLAB Function ==
  data: spring_torques input; R1 output; sample_time parameter; R2 output; R3 output; R4 output
function [R1, R2, R3, R4] = MeasurementCovariance(spring_torques, sample_time)
         
    high_torque_threshold = 80;
    low_torque_threshold = 50;
    high_deviation = 10;
    low_deviation = 0.1;
    
    deviation = (abs(spring_torques)-low_torque_threshold)*(low_deviation-high_deviation)/(high_torque_threshold-low_torque_threshold) + high_deviation;
    deviation(abs(spring_torques) <= low_torque_threshold) = high_deviation;
    deviation(abs(spring_torques) >= high_torque_threshold) = low_deviation;

    R1 = diag([(1e-6)^2, deviation(1)^2])/sample_time;
    R2 = diag([(1e-6)^2, deviation(2)^2])/sample_time;
    R3 = diag([(1e-6)^2, deviation(3)^2])/sample_time;
    R4 = diag([(1e-6)^2, deviation(4)^2])/sample_time;
end

== matlab function actuator_control/Misc/Detect Collision ==
  data: time input; spring_torque input; load_torque_derivative input; in_collision output; swing_collision_wait_time parameter
function in_collision = detect_collision(time, spring_torque, load_torque_derivative, swing_collision_wait_time)
    
    persistent collision_state time_of_collision;
    if isempty(collision_state)
        collision_state = logical(zeros(4,1));
        time_of_collision = zeros(4,1);
    end

    collision_detected = (abs(load_torque_derivative) > 2000 | abs(spring_torque) >= 50) & (time - time_of_collision > (1.5*swing_collision_wait_time));
    time_of_collision(collision_detected) = time;
    collision_state = collision_state | collision_detected;
    time_since_collision = time - time_of_collision;
    out_of_collision = (time_since_collision > swing_collision_wait_time) & (abs(spring_torque) < 50);
    collision_state(out_of_collision) = 0;
    %in_collision = collision_state;
    in_collision = [collision_state(1) | collision_state(2);
                    collision_state(1) | collision_state(2);
                    collision_state(3) | collision_state(4);
                    collision_state(3) | collision_state(4)];
    
end

== matlab function actuator_control/SEA Controller (Velocity Based)/Nonlinear Spring Force ==
  data: deflections input; tau_sea output
function tau_sea   = SeaSpringForce( deflections )
    tau_sea = SeaSpringForce( deflections );
end

== matlab function actuator_control/SEA Kalman Filter (swing)/Covariance Estimates ==
  data: absolute_motor input; absolute_load input; estimated_motor_velocity input; estimated_load_velocity input; time input; Q1 output; R1 output; Q2 output; R2 output; R_kalman_absolute_normal parameter; R_kalman_absolute_fail parameter; R_kalman_incremental_unloaded parameter; R_kalman_incremental_loaded parameter; kalman_load_to_deflect_transmission parameter; Q3 output; R3 output; Q4 output; R4 output; Q_kalman_load_torque parameter; Q_kalman_rotor_torque parameter; Q_kalman_trunk_torque parameter; sea_kalman_sample_time parameter; k_sea_low parameter; unfiltered_spring_torque output; sample_time parameter
function [Q1, R1, Q2, R2, Q3, R3, Q4, R4, unfiltered_spring_torque] = covariance( absolute_motor, absolute_load, estimated_motor_velocity, estimated_load_velocity, time,...
                                                        R_kalman_absolute_normal, R_kalman_absolute_fail, R_kalman_incremental_unloaded, R_kalman_incremental_loaded, ...
                                                        kalman_load_to_deflect_transmission, Q_kalman_load_torque, Q_kalman_rotor_torque, Q_kalman_trunk_torque, sea_kalman_sample_time, k_sea_low, sample_time)

    % Initialize persistent absolute measurement variables
    persistent previous_absolute_gear previous_absolute_load
    if isempty(previous_absolute_gear)
        previous_absolute_gear = absolute_motor;
    end
    if isempty(previous_absolute_load)
        previous_absolute_load = absolute_load;
    end
    
    % Measurement covariance
    time_past_medulla_reading = rem(time, sample_time);
    R_absolute_motor = ones(4,1)*R_kalman_absolute_normal + (time_past_medulla_reading*estimated_motor_velocity).^2;
    R_absolute_load = ones(4,1)*R_kalman_absolute_normal  + (time_past_medulla_reading*estimated_load_velocity).^2;
    dropped_out = previous_absolute_gear == absolute_motor;
   % R_absolute_motor(dropped_out) = R_kalman_absolute_fail;
    dropped_out = previous_absolute_load == absolute_load;
   % R_absolute_load(dropped_out) = R_kalman_absolute_fail;
    unfiltered_spring_torque = k_sea_low.*(absolute_motor - absolute_load);
    R_incremental_scale = min(abs(unfiltered_spring_torque)/kalman_load_to_deflect_transmission, 1);
    R_incremental = R_incremental_scale*R_kalman_incremental_loaded + (1-R_incremental_scale)*R_kalman_incremental_unloaded;
    R1 = diag([R_absolute_motor(1), R_incremental(1), R_absolute_load(1)])/sea_kalman_sample_time;
    R2 = diag([R_absolute_motor(2), R_incremental(2), R_absolute_load(2)])/sea_kalman_sample_time;
    R3 = diag([R_absolute_motor(3), R_incremental(3), R_absolute_load(3)])/sea_kalman_sample_time;
    R4 = diag([R_absolute_motor(4), R_incremental(4), R_absolute_load(4)])/sea_kalman_sample_time;
    
    % Process noise covariance
    Q1 = diag([Q_kalman_rotor_torque, Q_kalman_trunk_torque, Q_kalman_load_torque])*sea_kalman_sample_time;
    Q2 = diag([Q_kalman_rotor_torque, Q_kalman_trunk_torque, Q_kalman_load_torque])*sea_kalman_sample_time;
    Q3 = diag([Q_kalman_rotor_torque, Q_kalman_trunk_torque, Q_kalman_load_torque])*sea_kalman_sample_time;
    Q4 = diag([Q_kalman_rotor_torque, Q_kalman_trunk_torque, Q_kalman_load_torque])*sea_kalman_sample_time;

    previous_absolute_gear = absolute_motor;
    previous_absolute_load = absolute_load;
end

== matlab function actuator_control/SEA Kalman Filter (swing)/HarmonicDriveEfficiency ==
  data: motor_velocity input; mu output; load_torque input; N parameter
function mu = mu(motor_velocity, load_torque, N)
    rpm = motor_velocity*N*60/(2*pi);
    mu = HarmonicDriveEfficiency( rpm, load_torque );
end
